simulink model "noisy_observer"  (R2025b)
settings: Solver=VariableStepAuto  StartTime=0.0  StopTime=400  RelTol=1e-3
values from neighbouring files (symbols this model uses):
  A = [0 -0.0122335357927 0 0.04653303839 1 0 0 0 0 -2.91800139921 0 37.7525456689 ... (16 elements, 4x4)]    [matlab.mat]
  B = [0 -0.714154574773 0 -0.000498818992568]    [matlab.mat]
  C = [1 0 0 0 0 1 0 0 0 0 1 0 ... (16 elements, 4x4)]    [matlab.mat]
  K_lqr = [-1231.62178055 75.4404321566 -1810304.48785 -294623.729953]    [matlab.mat]
undefined symbols (not defined in the file or in its folder): a, b, K_kalman, x_0
libraries: simulink x1
settings Model: Creator=shree  LastModifiedBy=shree

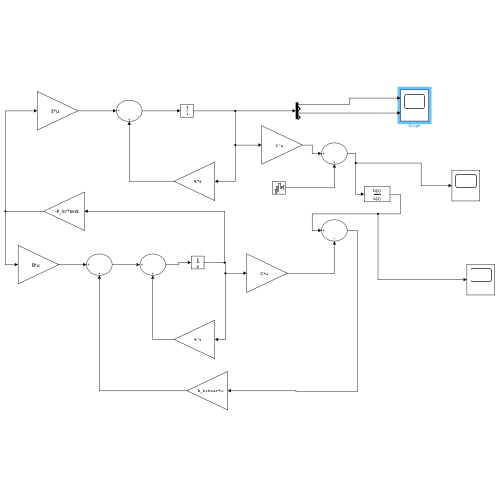
[thumbnail: Simulink's stored preview of the top-level diagram]
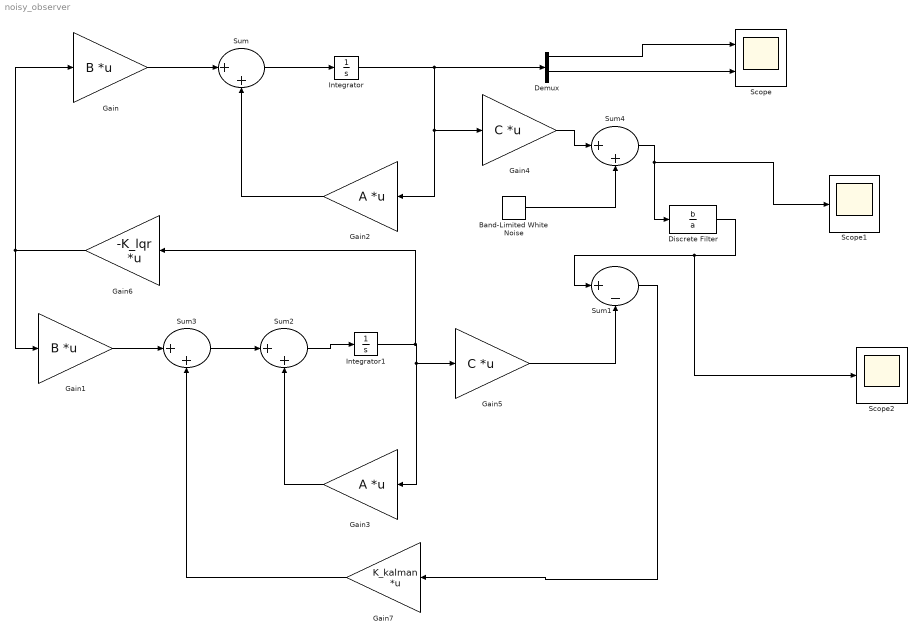
== system noisy_observer ==
  Band-Limited White Noise : simulink/Sources/Band-Limited White Noise  Cov=[0.000000000001]  Ts=0.00001  seed=[23341]
  Demux : Demux
  Discrete Filter : DiscreteFilter  Numerator=b  Denominator=a
  Gain : Gain  Gain=B  Multiplication=Matrix(K*u)
  Gain1 : Gain  Gain=B  Multiplication=Matrix(K*u)
  Gain2 : Gain  Gain=A  Multiplication=Matrix(K*u)
  Gain3 : Gain  Gain=A  Multiplication=Matrix(K*u)
  Gain4 : Gain  Gain=C  Multiplication=Matrix(K*u)
  Gain5 : Gain  Gain=C  Multiplication=Matrix(K*u)
  Gain6 : Gain  Gain=-K_lqr  Multiplication=Matrix(K*u) (u vector)
  Gain7 : Gain  Gain=K_kalman  Multiplication=Matrix(K*u)
  Integrator : Integrator  InitialCondition=x_0
  Integrator1 : Integrator  InitialCondition=[0.002, 0 , deg2rad(2),0]
  Scope : Scope  NumInputPorts=2
      settings: ActiveDisplayYMinimum=-0.1476589325826046  ActiveDisplayYMaximum=0.11895587776659461
  Scope1 : Scope
      settings: ActiveDisplayYMinimum=-0.14214609516866622  ActiveDisplayYMaximum=0.12446871518053282
  Scope2 : Scope
      settings: ActiveDisplayYMinimum=-0.14214609516866622  ActiveDisplayYMaximum=0.12446871518053282  DataLoggingVariableName=ScopeData2
  Sum{,2..4} (4 alike) : Sum  Inputs=|++
  Sum1 : Sum  Inputs=|+-
  wires:
  Integrator/1 -> Gain2/1, Gain4/1, Demux/1
  Sum3/1 -> Sum2/1
  Sum1/1 -> Gain7/1
  Sum/1 -> Integrator/1
  Integrator1/1 -> Gain6/1, Gain3/1, Gain5/1
  Demux/1 -> Scope/1
  Gain1/1 -> Sum3/1
  Gain3/1 -> Sum2/2
  Sum2/1 -> Integrator1/1
  Gain5/1 -> Sum1/2
  Gain6/1 -> Gain/1, Gain1/1
  Gain2/1 -> Sum/2
  Gain7/1 -> Sum3/2
  Gain/1 -> Sum/1
  Gain4/1 -> Sum4/1
  Band-Limited White Noise/1 -> Sum4/2
  Sum4/1 -> Scope1/1, Discrete Filter/1
  Discrete Filter/1 -> Scope2/1, Sum1/1
  Demux/3 -> Scope/2
